simulink model "Pacemaker_A1_full"  (R2022b)
settings: Solver=FixedStepAuto  StartTime=0.0  StopTime=10.0  FixedStep=1e-3  RelTol=1e-3  EnableMultiTasking=on
undefined symbols (not defined in the file): D0, D1, D10, D11, D12, D13, D2, D3, D5, D6, D8, D9, PTA0, PTA1, PTA2, PTB9, PTC16, PTC17, PTC2, PTC4, PTD0, PTD1, PTD2, PTD3
libraries: frdmk64flib x14
settings Model: ExtModeTrigDuration=5  Creator=27161  LastModifiedBy=27161
settings SolverCC: AlgebraicLoopSolver=TrustRegion
settings OptimizationCC: EnhancedBackFolding=on  PassReuseOutputArgsAs=Individual arguments  ZeroExternalMemoryAtStartup=off  ZeroInternalMemoryAtStartup=off  MaxStackSize=64  OptimizeBlockOrder=speed  DifferentSizesBufferReuse=on  OptimizationCustomize=off  EfficientTunableParamExpr=on
settings DebuggingCC: ParameterTunabilityLossMsg=error  UnconnectedInputMsg=warning  UnconnectedOutputMsg=warning  UnconnectedLineMsg=warning  SFMachineParentedDataDiag=warning
settings HardwareCC: ProdBitPerPointer=32  ProdBitPerSizeT=32  ProdBitPerPtrDiffT=32  ProdLargestAtomicInteger=Long  ProdLargestAtomicFloat=Double  ProdWordSize=32  ProdHWDeviceType=ARM Compatible->ARM Cortex
settings ModelReferenceCC: EnableRefExpFcnMdlSchedulingChecks=on
settings SFSimCC: MATLABDynamicMemAlloc=off
settings RTWCC: Description=Embedded Coder  SystemTargetFile=ert.tlc  HardwareBoard=NXP FRDM-K64F  TLCOptions="-aInlineSetEventsForThisBaseRateFcn=TLC_FALSE -aSuppressMultiTaskScheduler=TLC_FALSE  -aRateBasedStepFcn=0"  TemplateMakefile=ert_default_tmf  Toolchain=GNU Tools for ARM Embedded Processors
settings CodeAppCC: ForceParamTrailComments=on  IgnoreCustomStorageClasses=off  OperatorAnnotations=on  SimulinkDataObjDesc=on  SFDataObjDesc=on  InsertBlockDesc=on

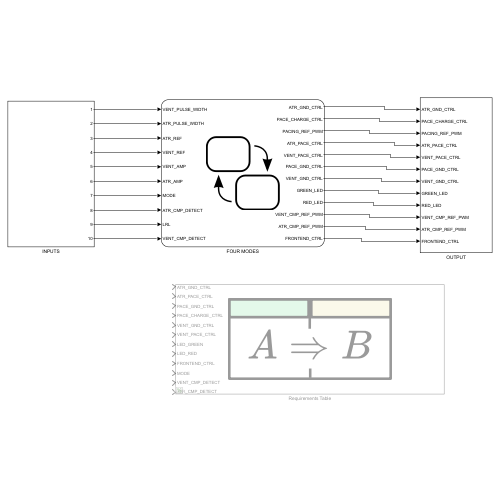
[thumbnail: Simulink's stored preview of the top-level diagram]
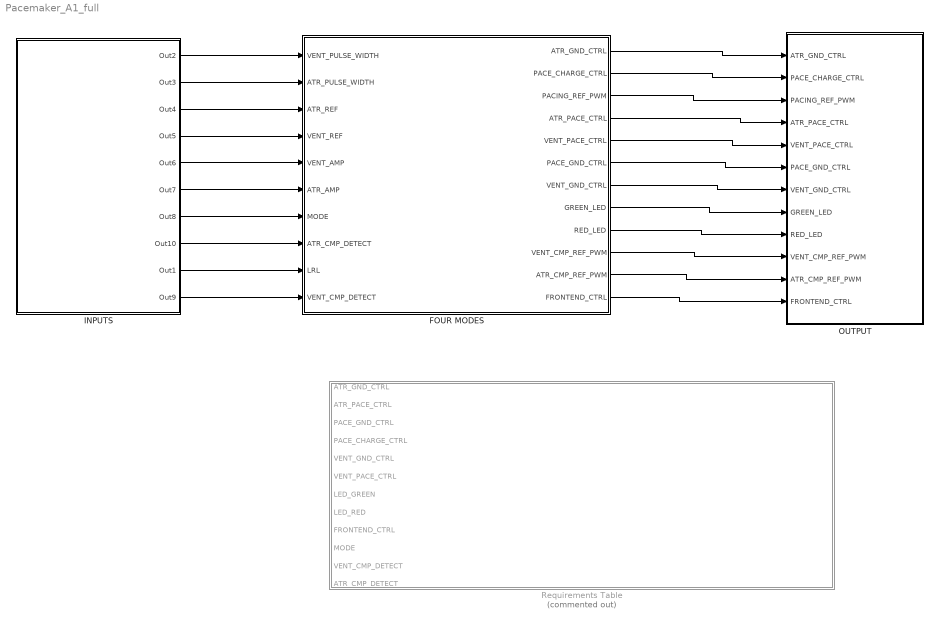
== system Pacemaker_A1_full ==
  FOUR MODES : Stateflow chart  TreatAsAtomicUnit=on
      settings: PortSchema="{\"entries\":[{\"content\":{\"sides\":[{\"content\":{\"connectorIds\":[\"In2\",\"In1\",\"In6\",\"In3\",\"In5\",\"In7\",\"In8\",\"In9\",\"In10\",\"In4\"]},\"type\":\"ConnectorPlacement.EquallySpacedRectSide\",\"uuid\":\"6661be6b-aedb-4592-878a-fd9116f5820d\"},{\"content\":{\"connectorIds\":[\"Out7\",\"Out1\",\"Out2\",\"Out3\",\"Out4\",\"Out6\",\"Out5\",\"Out9\",\"Out10\",\"Out11\",\"Out12\",\"Out8\"],\"side\":\"RIGHT\"},\"type\":\"ConnectorPlacement.EquallySpacedRectSide\",\"uuid\":\"f16586c3-0c99-4971-ba5f-75b93d25059c\"},{\"content\":{\"connectorIds\":[],\"side\":\"TOP\"},\"type\":\"ConnectorPlacement.EquallySpacedRectSide\",\"uuid\":\"27cb1bd0-c170-4ecc-a4df-3797e7aecef3\"}]},\"type\":\"ConnectorPlacement.EquallySpacedConnector\",\"uuid\":\"03557791-41f4-4916-8cde-1fcab0cf663d\"}],\"packageUris\":[\"http://schema.mathworks.com/mf0/Connector/R2020b\"],\"version\":\"1.0\"}"
  INPUTS : Subsystem
  OUTPUT : Subsystem
  Requirements Table : Requirements Table  Commented=on  TreatAsAtomicUnit=on
  wires:
  FOUR MODES/7(ATR_GND_CTRL) -> OUTPUT/1(ATR_GND_CTRL)
  FOUR MODES/1(PACE_CHARGE_CTRL) -> OUTPUT/2(PACE_CHARGE_CTRL)
  FOUR MODES/2(PACING_REF_PWM) -> OUTPUT/3(PACING_REF_PWM)
  FOUR MODES/3(ATR_PACE_CTRL) -> OUTPUT/4(ATR_PACE_CTRL)
  FOUR MODES/4(VENT_PACE_CTRL) -> OUTPUT/5(VENT_PACE_CTRL)
  FOUR MODES/5(VENT_GND_CTRL) -> OUTPUT/7(VENT_GND_CTRL)
  FOUR MODES/6(PACE_GND_CTRL) -> OUTPUT/6(PACE_GND_CTRL)
  INPUTS/1(Out2) -> FOUR MODES/2(VENT_PULSE_WIDTH)
  INPUTS/2(Out3) -> FOUR MODES/1(ATR_PULSE_WIDTH)
  INPUTS/3(Out4) -> FOUR MODES/6(ATR_REF)
  INPUTS/4(Out5) -> FOUR MODES/3(VENT_REF)
  INPUTS/5(Out6) -> FOUR MODES/5(VENT_AMP)
  INPUTS/7(Out8) -> FOUR MODES/8(MODE)
  INPUTS/6(Out7) -> FOUR MODES/7(ATR_AMP)
  FOUR MODES/9(GREEN_LED) -> OUTPUT/8(GREEN_LED)
  FOUR MODES/12(ATR_CMP_REF_PWM) -> OUTPUT/11(ATR_CMP_REF_PWM)
  FOUR MODES/11(VENT_CMP_REF_PWM) -> OUTPUT/10(VENT_CMP_REF_PWM)
  FOUR MODES/10(RED_LED) -> OUTPUT/9(RED_LED)
  FOUR MODES/8(FRONTEND_CTRL) -> OUTPUT/12(FRONTEND_CTRL)
  INPUTS/8(Out10) -> FOUR MODES/9(ATR_CMP_DETECT)
  INPUTS/10(Out9) -> FOUR MODES/4(VENT_CMP_DETECT)
  INPUTS/9(Out1) -> FOUR MODES/10(LRL)

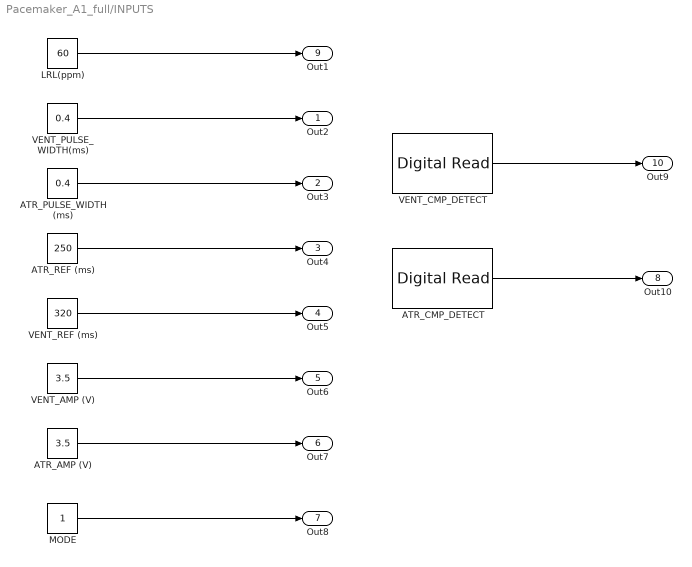
== system Pacemaker_A1_full/INPUTS ==
  ATR_AMP (V) : Constant  Value=3.5
  ATR_CMP_DETECT : frdmk64flib/Digital Read  Whichpin=PTC16 (D0)  SampleTime=-1
  ATR_PULSE_WIDTH (ms) : Constant  Value=0.4
  ATR_REF (ms) : Constant  Value=250
  LRL(ppm) : Constant  Value=60
  MODE : Constant
  VENT_AMP (V) : Constant  Value=3.5
  VENT_CMP_DETECT : frdmk64flib/Digital Read  Whichpin=PTC17 (D1)  SampleTime=-1
  VENT_PULSE_WIDTH(ms) : Constant  Value=0.4
  VENT_REF (ms) : Constant  Value=320
  Out2 : Outport
  Out3 : Outport  Port=2
  Out4 : Outport  Port=3
  Out5 : Outport  Port=4
  Out6 : Outport  Port=5
  Out7 : Outport  Port=6
  Out8 : Outport  Port=7
  Out10 : Outport  Port=8
  Out1 : Outport  Port=9
  Out9 : Outport  Port=10
  wires:
  LRL(ppm)/1 -> Out1/1
  VENT_PULSE_WIDTH(ms)/1 -> Out2/1
  ATR_PULSE_WIDTH (ms)/1 -> Out3/1
  ATR_REF (ms)/1 -> Out4/1
  VENT_REF (ms)/1 -> Out5/1
  VENT_AMP (V)/1 -> Out6/1
  ATR_AMP (V)/1 -> Out7/1
  MODE/1 -> Out8/1
  ATR_CMP_DETECT/1 -> Out10/1
  VENT_CMP_DETECT/1 -> Out9/1

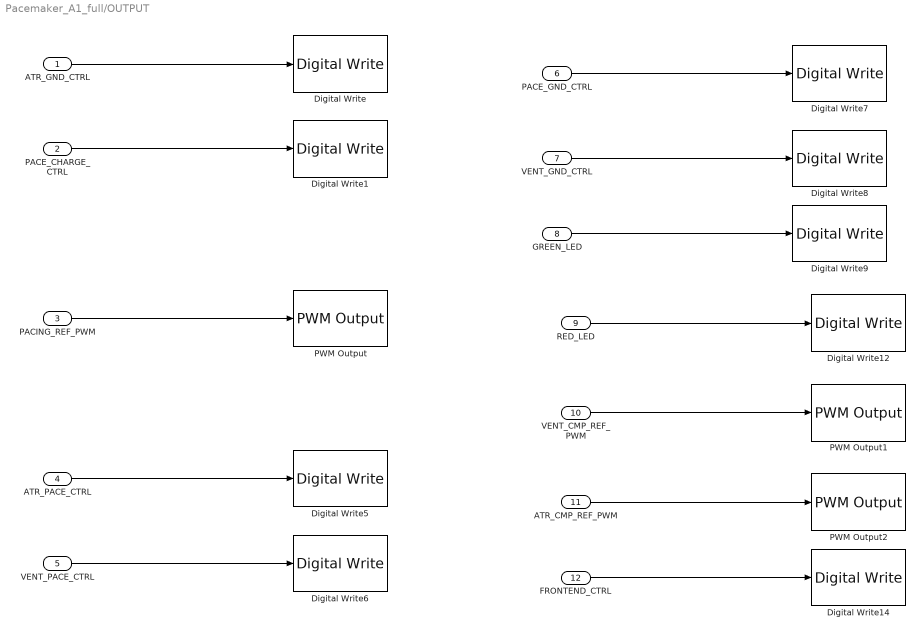
== system Pacemaker_A1_full/OUTPUT ==
  ATR_GND_CTRL : Inport
  PACE_CHARGE_CTRL : Inport  Port=2
  PACING_REF_PWM : Inport  Port=3
  ATR_PACE_CTRL : Inport  Port=4
  VENT_PACE_CTRL : Inport  Port=5
  PACE_GND_CTRL : Inport  Port=6
  VENT_GND_CTRL : Inport  Port=7
  GREEN_LED : Inport  Port=8
  RED_LED : Inport  Port=9
  VENT_CMP_REF_PWM : Inport  Port=10
  ATR_CMP_REF_PWM : Inport  Port=11
  FRONTEND_CTRL : Inport  Port=12
  Digital Write : frdmk64flib/Digital Write  Whichpin=PTD2 (D11)
  Digital Write1 : frdmk64flib/Digital Write  Whichpin=PTB9 (D2)
  Digital Write12 : frdmk64flib/Digital Write  Whichpin=RED_LED
  Digital Write14 : frdmk64flib/Digital Write  Whichpin=PTD1 (D13)
  Digital Write5 : frdmk64flib/Digital Write  Whichpin=PTA0 (D8)
  Digital Write6 : frdmk64flib/Digital Write  Whichpin=PTC4 (D9)
  Digital Write7 : frdmk64flib/Digital Write  Whichpin=PTD0 (D10)
  Digital Write8 : frdmk64flib/Digital Write  Whichpin=PTD3 (D12)
  Digital Write9 : frdmk64flib/Digital Write  Whichpin=GREEN_LED
  PWM Output : frdmk64flib/PWM Output  Whichpin=PTA2 (D5)  InitialFrequency=2000  InitialDutyCycle=0
  PWM Output1 : frdmk64flib/PWM Output  Whichpin=PTA1 (D3)  InitialFrequency=2000  InitialDutyCycle=0
  PWM Output2 : frdmk64flib/PWM Output  Whichpin=PTC2 (D6)  InitialFrequency=2000  InitialDutyCycle=0
  wires:
  ATR_GND_CTRL/1 -> Digital Write/1
  PACE_CHARGE_CTRL/1 -> Digital Write1/1
  PACING_REF_PWM/1 -> PWM Output/1
  ATR_PACE_CTRL/1 -> Digital Write5/1
  VENT_PACE_CTRL/1 -> Digital Write6/1
  PACE_GND_CTRL/1 -> Digital Write7/1
  VENT_GND_CTRL/1 -> Digital Write8/1
  GREEN_LED/1 -> Digital Write9/1
  ATR_CMP_REF_PWM/1 -> PWM Output2/1
  VENT_CMP_REF_PWM/1 -> PWM Output1/1
  RED_LED/1 -> Digital Write12/1
  FRONTEND_CTRL/1 -> Digital Write14/1

== stateflow chart Pacemaker_A1_full/Requirements Table ==
  (default) -> (junction 1073751917)
  (junction 1073751917) -> (junction 1073751918) : {
      | % SF_REQ_REV_07
      | }
  (junction 1073751918) -> (junction 1073751920) : {
      | % HEADER_ASSIGNMENTS
      |
      | }
  (junction 1073751920) -> (junction 1073751922) : {
      | % START_A_4
      | }
  (junction 1073751922) -> (junction 1073751924) : {
      | }
  (junction 1073751924) -> (junction 1073751926)
  (junction 1073751926) -> (junction 1073751928) : {
      | }
  (junction 1073751928) -> (junction 1073751930) : {
      | % END_A_4
      | }
  (junction 1073751930) -> (junction 1073751932) : {
      | % START_R_1
      | }
  (junction 1073751932) -> (junction 1073751934) : {
      | }
  (junction 1073751934) -> (junction 1073751936)
  (junction 1073751936) -> (junction 1073751938) [order 1] : [(((MODE) == (1)))]
  (junction 1073751936) -> (junction 1073751980) [order 2]
  (junction 1073751938) -> (junction 1073751940) : {
      |
      |
      | }
  (junction 1073751940) -> (junction 1073751942) : {
      | }
  (junction 1073751942) -> (junction 1073751944) : {
      | % START_R_7
      | }
  (junction 1073751944) -> (junction 1073751946) : {
      | }
  (junction 1073751946) -> (junction 1073751948)
  (junction 1073751948) -> (junction 1073751950) [order 1] : [(((state) == (1)))]
  (junction 1073751948) -> (junction 1073751956) [order 2]
  (junction 1073751950) -> (junction 1073751952) : {
      | reqtable_postcondition((((PACE_GND_CTRL) == (true))) && (((PACE_CHARGE_CTRL) == (false))) && (((ATR_GND_CTRL) == (false))) && (((ATR_PACE_CTRL) == (true))) && (((LED_GREEN) == (false))), 'R:1.1');
      |
      |
      | }
  (junction 1073751952) -> (junction 1073751954) : {
      | }
  (junction 1073751954) -> (junction 1073751956)
  (junction 1073751956) -> (junction 1073751958)
  (junction 1073751958) -> (junction 1073751960) : {
      | % END_R_7
      | }
  (junction 1073751960) -> (junction 1073751962) : {
      | % START_R_34
      | }
  (junction 1073751962) -> (junction 1073751964) : {
      | }
  (junction 1073751964) -> (junction 1073751966)
  (junction 1073751966) -> (junction 1073751968) [order 1] : [(((state) == (2)))]
  (junction 1073751966) -> (junction 1073751974) [order 2]
  (junction 1073751968) -> (junction 1073751970) : {
      | reqtable_postcondition((((PACE_GND_CTRL) == (true))) && (((PACE_CHARGE_CTRL) == (true))) && (((ATR_GND_CTRL) == (true))) && (((ATR_PACE_CTRL) == (false))) && (((LED_GREEN) == (true))), 'R:1.2');
      |
      |
      | }
  (junction 1073751970) -> (junction 1073751972) : {
      | }
  (junction 1073751972) -> (junction 1073751974)
  (junction 1073751974) -> (junction 1073751976)
  (junction 1073751976) -> (junction 1073751978) : {
      | % END_R_34
      | }
  (junction 1073751978) -> (junction 1073751980)
  (junction 1073751980) -> (junction 1073751982)
  (junction 1073751982) -> (junction 1073751984) : {
      | % END_R_1
      | }
  (junction 1073751984) -> (junction 1073751986) : {
      | % START_R_10
      | }
  (junction 1073751986) -> (junction 1073751988) : {
      | }
  (junction 1073751988) -> (junction 1073751990)
  (junction 1073751990) -> (junction 1073751992) [order 1] : [(((MODE) == (2)))]
  (junction 1073751990) -> (junction 1073752034) [order 2]
  (junction 1073751992) -> (junction 1073751994) : {
      |
      |
      | }
  (junction 1073751994) -> (junction 1073751996) : {
      | }
  (junction 1073751996) -> (junction 1073751998) : {
      | % START_R_28
      | }
  (junction 1073751998) -> (junction 1073752000) : {
      | }
  (junction 1073752000) -> (junction 1073752002)
  (junction 1073752002) -> (junction 1073752004) [order 1] : [(((state) == (1)))]
  (junction 1073752002) -> (junction 1073752010) [order 2]
  (junction 1073752004) -> (junction 1073752006) : {
      | reqtable_postcondition((((PACE_GND_CTRL) == (true))) && (((PACE_CHARGE_CTRL) == (false))) && (((VENT_PACE_CTRL) == (true))) && (((VENT_GND_CTRL) == (false))) && (((LED_RED) == (false))), 'R:2.1');
      |
      |
      | }
  (junction 1073752006) -> (junction 1073752008) : {
      | }
  (junction 1073752008) -> (junction 1073752010)
  (junction 1073752010) -> (junction 1073752012)
  (junction 1073752012) -> (junction 1073752014) : {
      | % END_R_28
      | }
  (junction 1073752014) -> (junction 1073752016) : {
      | % START_R_31
      | }
  (junction 1073752016) -> (junction 1073752018) : {
      | }
  (junction 1073752018) -> (junction 1073752020)
  (junction 1073752020) -> (junction 1073752022) [order 1] : [(((state) == (2)))]
  (junction 1073752020) -> (junction 1073752028) [order 2]
  (junction 1073752022) -> (junction 1073752024) : {
      | reqtable_postcondition((((PACE_GND_CTRL) == (true))) && (((PACE_CHARGE_CTRL) == (true))) && (((VENT_PACE_CTRL) == (false))) && (((VENT_GND_CTRL) == (true))) && (((LED_RED) == (true))), 'R:2.2');
      |
      |
      | }
  (junction 1073752024) -> (junction 1073752026) : {
      | }
  (junction 1073752026) -> (junction 1073752028)
  (junction 1073752028) -> (junction 1073752030)
  (junction 1073752030) -> (junction 1073752032) : {
      | % END_R_31
      | }
  (junction 1073752032) -> (junction 1073752034)
  (junction 1073752034) -> (junction 1073752036)
  (junction 1073752036) -> (junction 1073752038) : {
      | % END_R_10
      | }
  (junction 1073752038) -> (junction 1073752040) : {
      | % START_R_13
      | }
  (junction 1073752040) -> (junction 1073752042) : {
      | }
  (junction 1073752042) -> (junction 1073752044)
  (junction 1073752044) -> (junction 1073752046) [order 1] : [(((MODE) == (3)))]
  (junction 1073752044) -> (junction 1073752106) [order 2]
  (junction 1073752046) -> (junction 1073752048) : {
      |
      |
      | }
  (junction 1073752048) -> (junction 1073752050) : {
      | }
  (junction 1073752050) -> (junction 1073752052) : {
      | % START_R_19
      | }
  (junction 1073752052) -> (junction 1073752054) : {
      | }
  (junction 1073752054) -> (junction 1073752056)
  (junction 1073752056) -> (junction 1073752058) [order 1] : [(((state) == (1)))]
  (junction 1073752056) -> (junction 1073752064) [order 2]
  (junction 1073752058) -> (junction 1073752060) : {
      | reqtable_postcondition((((PACE_GND_CTRL) == (true))) && (((PACE_CHARGE_CTRL) == (true))) && (((VENT_PACE_CTRL) == (false))) && (((VENT_GND_CTRL) == (true))) && (((FRONTEND_CTRL) == (true))) && (((LED_RED) == (true))), 'R:3.1');
      |
      |
      | }
  (junction 1073752060) -> (junction 1073752062) : {
      | }
  (junction 1073752062) -> (junction 1073752064)
  (junction 1073752064) -> (junction 1073752066)
  (junction 1073752066) -> (junction 1073752068) : {
      | % END_R_19
      | }
  (junction 1073752068) -> (junction 1073752070) : {
      | % START_R_22
      | }
  (junction 1073752070) -> (junction 1073752072) : {
      | }
  (junction 1073752072) -> (junction 1073752074)
  (junction 1073752074) -> (junction 1073752076) [order 1] : [(((state) == (2)))]
  (junction 1073752074) -> (junction 1073752082) [order 2]
  (junction 1073752076) -> (junction 1073752078) : {
      | reqtable_postcondition((((PACE_GND_CTRL) == (true))) && (((PACE_CHARGE_CTRL) == (false))) && (((VENT_PACE_CTRL) == (true))) && (((VENT_GND_CTRL) == (false))) && (((LED_GREEN) == (true))), 'R:3.2');
      |
      |
      | }
  (junction 1073752078) -> (junction 1073752080) : {
      | }
  (junction 1073752080) -> (junction 1073752082)
  (junction 1073752082) -> (junction 1073752084)
  (junction 1073752084) -> (junction 1073752086) : {
      | % END_R_22
      | }
  (junction 1073752086) -> (junction 1073752088) : {
      | % START_R_43
      | }
  (junction 1073752088) -> (junction 1073752090) : {
      | }
  (junction 1073752090) -> (junction 1073752092)
  (junction 1073752092) -> (junction 1073752094) [order 1] : [(((state) == (3)))]
  (junction 1073752092) -> (junction 1073752100) [order 2]
  (junction 1073752094) -> (junction 1073752096) : {
      | reqtable_postcondition((((PACE_GND_CTRL) == (true))) && (((PACE_CHARGE_CTRL) == (false))) && (((VENT_PACE_CTRL) == (false))) && (((VENT_GND_CTRL) == (true))) && (((FRONTEND_CTRL) == (false))) && (((LED_RED) == (false))), 'R:3.3');
      |
      |
      | }
  (junction 1073752096) -> (junction 1073752098) : {
      | }
  (junction 1073752098) -> (junction 1073752100)
  (junction 1073752100) -> (junction 1073752102)
  (junction 1073752102) -> (junction 1073752104) : {
      | % END_R_43
      | }
  (junction 1073752104) -> (junction 1073752106)
  (junction 1073752106) -> (junction 1073752108)
  (junction 1073752108) -> (junction 1073752110) : {
      | % END_R_13
      | }
  (junction 1073752110) -> (junction 1073752112) : {
      | % START_R_16
      | }
  (junction 1073752112) -> (junction 1073752114) : {
      | }
  (junction 1073752114) -> (junction 1073752116)
  (junction 1073752116) -> (junction 1073752118) [order 1] : [(((MODE) == (4)))]
  (junction 1073752116) -> (junction 1073752178) [order 2]
  (junction 1073752118) -> (junction 1073752120) : {
      |
      |
      | }
  (junction 1073752120) -> (junction 1073752122) : {
      | }
  (junction 1073752122) -> (junction 1073752124) : {
      | % START_R_37
      | }
  (junction 1073752124) -> (junction 1073752126) : {
      | }
  (junction 1073752126) -> (junction 1073752128)
  (junction 1073752128) -> (junction 1073752130) [order 1] : [(((state) == (1)))]
  (junction 1073752128) -> (junction 1073752136) [order 2]
  (junction 1073752130) -> (junction 1073752132) : {
      | reqtable_postcondition((((PACE_GND_CTRL) == (true))) && (((PACE_CHARGE_CTRL) == (true))) && (((ATR_GND_CTRL) == (true))) && (((ATR_PACE_CTRL) == (false))) && (((FRONTEND_CTRL) == (true))) && (((LED_GREEN) == (true))), 'R:4.1');
      |
      |
      | }
  (junction 1073752132) -> (junction 1073752134) : {
      | }
  (junction 1073752134) -> (junction 1073752136)
  (junction 1073752136) -> (junction 1073752138)
  (junction 1073752138) -> (junction 1073752140) : {
      | % END_R_37
      | }
  (junction 1073752140) -> (junction 1073752142) : {
      | % START_R_40
      | }
  (junction 1073752142) -> (junction 1073752144) : {
      | }
  (junction 1073752144) -> (junction 1073752146)
  (junction 1073752146) -> (junction 1073752148) [order 1] : [(((state) == (2)))]
  (junction 1073752146) -> (junction 1073752154) [order 2]
  (junction 1073752148) -> (junction 1073752150) : {
      | reqtable_postcondition((((PACE_GND_CTRL) == (true))) && (((PACE_CHARGE_CTRL) == (false))) && (((ATR_GND_CTRL) == (false))) && (((ATR_PACE_CTRL) == (true))) && (((LED_RED) == (true))), 'R:4.2');
      |
      |
      | }
  (junction 1073752150) -> (junction 1073752152) : {
      | }
  (junction 1073752152) -> (junction 1073752154)
  (junction 1073752154) -> (junction 1073752156)
  (junction 1073752156) -> (junction 1073752158) : {
      | % END_R_40
      | }
  (junction 1073752158) -> (junction 1073752160) : {
      | % START_R_46
      | }
  (junction 1073752160) -> (junction 1073752162) : {
      | }
  (junction 1073752162) -> (junction 1073752164)
  (junction 1073752164) -> (junction 1073752166) [order 1] : [(((state) == (3)))]
  (junction 1073752164) -> (junction 1073752172) [order 2]
  (junction 1073752166) -> (junction 1073752168) : {
      | reqtable_postcondition((((PACE_GND_CTRL) == (true))) && (((PACE_CHARGE_CTRL) == (false))) && (((ATR_GND_CTRL) == (true))) && (((ATR_PACE_CTRL) == (false))) && (((FRONTEND_CTRL) == (false))) && (((LED_GREEN) == (false))), 'R:4.3');
      |
      |
      | }
  (junction 1073752168) -> (junction 1073752170) : {
      | }
  (junction 1073752170) -> (junction 1073752172)
  (junction 1073752172) -> (junction 1073752174)
  (junction 1073752174) -> (junction 1073752176) : {
      | % END_R_46
      | }
  (junction 1073752176) -> (junction 1073752178)
  (junction 1073752178) -> (junction 1073752180)
  (junction 1073752180) -> (junction 1073752182) : {
      | % END_R_16
      | }
  data: ATR_GND_CTRL input; ATR_PACE_CTRL input; PACE_GND_CTRL input; PACE_CHARGE_CTRL input; VENT_GND_CTRL input; VENT_PACE_CTRL input; LED_GREEN input; LED_RED input; FRONTEND_CTRL input; MODE input; VENT_CMP_DETECT input; ATR_CMP_DETECT input

== stateflow chart Pacemaker_A1_full/FOUR MODES ==
  note: In the pacing state, we connect C22 to C21 to pace the Atrium.
  note: In the AOO initial state, we start charging C22 to prepare to pace.
      | Also, we begin to discharge C21 from the last pace.
  state AOO_INITIAL
    entry:
    ATR_PACE_CTRL = false;
    ATR_GND_CTRL = true;
    PACE_CHARGE_CTRL = true;
    PACE_GND_CTRL = true;
    PACING_REF_PWM = ATR_AMP*20
    GREEN_LED = 1;
  state AOO_PACING
    PACE_CHARGE_CTRL = false;
    PACE_GND_CTRL = true;
    ATR_PACE_CTRL = true;
    ATR_GND_CTRL = false;
    GREEN_LED =0;
  note: In the MainState, we set all of our set points to 0 and detect which mode we go next.
  note: In the initial state of AAI, we have
      | sensor on to detact if the input voltage is higher
      | than our set threshlod.
      |
      | We also charge C22 for possible pacing
      | state happen when not detection of natural
      | pulse, and discharge C21 to end the pacing state.
      |
      | LED light is off at initial state.
  state MainState
    entry:
    ATR_PACE_CTRL = false;
    ATR_GND_CTRL = false;
    VENT_GND_CTRL = false;
    VENT_PACE_CTRL = false;
    PACE_CHARGE_CTRL = false;
    PACE_GND_CTRL = false;
    FRONTEND_CTRL = false;
  note: We have a total cycle of 60s/LRL(BPM)
  note: In the pacing state, we connect C22 to C21 to pace the Atrium
  state VOO_INITIAL
    entry:
    VENT_GND_CTRL = true;
    VENT_PACE_CTRL = false;
    PACE_CHARGE_CTRL = true;
    PACE_GND_CTRL = true;
    PACING_REF_PWM = VENT_AMP*20
    RED_LED = 1;
  state VOO_PACING
    PACE_CHARGE_CTRL = false;
    PACE_GND_CTRL = true;
    VENT_GND_CTRL = false;
    VENT_PACE_CTRL = true;
    RED_LED =0;
  state AAI_INITIAL
    entry:
    FRONTEND_CTRL= true;
    ATR_PACE_CTRL = false;
    PACING_REF_PWM = ATR_AMP/5*100;
    PACE_CHARGE_CTRL = true;
    PACE_GND_CTRL = true;
    ATR_GND_CTRL = true;
    ATR_CMP_REF_PWM = ATR_AMP/5*100;
    GREEN_LED = 1;
  note: In the VOO initial state, we start charging C22 to prepare to pace.
      | Also, we begin to discharge C21 from the last pace.
  note: After a pulse width, stop pacing
  note: When no detect natural pulse, pace the atrium
      | with connecting C22 to C11. Then wait for 1 cycle.
  state AAI_PACING
    entry:
    PACE_CHARGE_CTRL = false;
    PACE_GND_CTRL = true;
    ATR_PACE_CTRL = true;
    ATR_GND_CTRL = false;
    RED_LED = 1;
  note: In the Refractory state, sensor turn off.
      | A signal of this happen will have red LED turn on.
      | After a refractory period, go back to initial state.
  state AAI_REF
    entry:
    FRONTEND_CTRL = false;
    ATR_PACE_CTRL = false;
    ATR_GND_CTRL = true;
    ATR_CMP_REF_PWM = ATR_AMP*20;
    PACE_CHARGE_CTRL = false;
    PACE_GND_CTRL = true;
    GREEN_LED = 0;
  state VVI_REF
    entry:
    FRONTEND_CTRL = false;
    VENT_PACE_CTRL = false;
    VENT_GND_CTRL = true;
    PACING_REF_PWM = VENT_AMP*20;
    PACE_CHARGE_CTRL = false;
    PACE_GND_CTRL = true;
    RED_LED = 0;
  state VVI_INITIAL
    entry:
    PACING_REF_PWM = VENT_AMP*20;
    PACE_GND_CTRL = true;
    VENT_GND_CTRL = true;
    VENT_PACE_CTRL = false;
    PACE_CHARGE_CTRL = true;
    VENT_CMP_REF_PWM = VENT_AMP*20;
    FRONTEND_CTRL= true;
    RED_LED = 1;
  note: In the initial state of VVI, we turn the
      | sensor on to detect if the input voltage is higher
      | than our set threshlod.
      |
      | We also charge C22 for possible pacing
      | state happen when not detection of natural
      | pulse, and discharge C21 to end the pacing state.
      |
      | LED light is off at initial state.
  note: In the Refractory state, sensor turn off.
      | A signal of this happen will have red LED turn on.
      | After a refractory period, go back to initial state.
  state VVI_PACING
    entry:
    PACE_CHARGE_CTRL = false;
    PACE_GND_CTRL = true;
    VENT_GND_CTRL = false;
    VENT_PACE_CTRL = true;
    GREEN_LED = 1;
  note: Discharging C22 to C21 to pace the ventricle.
      | Same as VOO pacing.
  AOO_PACING -> AOO_INITIAL : [after(ATR_PULSE_WIDTH,msec)]
  (default) -> MainState [order 1]
  MainState -> AOO_INITIAL [order 1] : [MODE == 1]
  AOO_INITIAL -> AOO_PACING : [after(60000/LRL - ATR_PULSE_WIDTH,msec)]
  MainState -> AAI_INITIAL [order 4] : [MODE == 4]
  (default) -> AAI_INITIAL [order 2]
  VOO_INITIAL -> VOO_PACING : [after(60000/LRL - VENT_PULSE_WIDTH,msec)]
  MainState -> VVI_INITIAL [order 3] : [MODE == 3]
  MainState -> VOO_INITIAL [order 2] : [MODE == 2]
  VOO_PACING -> VOO_INITIAL : [after(VENT_PULSE_WIDTH,msec)]
  AAI_INITIAL -> AAI_PACING [order 1] : [(ATR_CMP_DETECT == false) && after(60000/LRL - ATR_PULSE_WIDTH - ATR_REF,msec)]
  AAI_INITIAL -> AAI_REF [order 2] : [ATR_CMP_DETECT == true]
  AAI_REF -> AAI_INITIAL : [after(ATR_REF, msec)]
  AAI_PACING -> AAI_REF : [after(ATR_PULSE_WIDTH,msec)]
  VVI_REF -> VVI_INITIAL : [after(VENT_REF, msec)]
  VVI_INITIAL -> VVI_REF [order 2] : [VENT_CMP_DETECT == 1]
  VVI_PACING -> VVI_REF : [after(VENT_PULSE_WIDTH,msec)]
  VVI_INITIAL -> VVI_PACING [order 1] : [(VENT_CMP_DETECT == 0) && after(60000/LRL - VENT_PULSE_WIDTH - VENT_REF,msec)]
  data: PACE_CHARGE_CTRL output; PACING_REF_PWM output; ATR_PACE_CTRL output; VENT_PACE_CTRL output; VENT_GND_CTRL output; PACE_GND_CTRL output; ATR_GND_CTRL output; ATR_PULSE_WIDTH input; VENT_PULSE_WIDTH input; FRONTEND_CTRL output; GREEN_LED output; VENT_REF input; VENT_CMP_DETECT input; VENT_AMP input; ATR_REF input; RED_LED output; ATR_AMP input; MODE input; VENT_CMP_REF_PWM output; ATR_CMP_DETECT input; ATR_CMP_REF_PWM output; LRL input
